simulink model "sschdlexThreePhaseConverterWithGridExample"  (R2023b)
settings: Solver=FixedStepDiscrete  StartTime=0  StopTime=0.09  RelTol=1e-3
InitFcn:
  | % LC filter parameters
  | 
  | Lf = 2e-3;
  | Rf = 20e-3;
  | Cf = 1e-6;
  | 
  | % Sample step size
  | 
  | % if ~exist('Tbase')
  |     Tbase = 5e-9;
  | % end
  | 
  | Ts = 1e-6;
  | Tsc=5e-5;
  | fsw = 10e3;
  | 
  | % PWM oversampling
  | oversampling = Ts/Tbase;
  | 
  | % Frame size for data transfer to CPU
  | frame_size = round(Tsc/Ts);
  | 
  | % Control constants
  | 
  | Kp_id = 1.5;
  | Ki_id = 400;
  | Kp_iq = 1.5;
  | Ki_iq = 400;
libraries: simulink x51, hdlsllib x23, fl_lib x15, nesl_utility x15, slrealtimeloglib x12, ee_lib x11, eeTransforms x3, slpidlib x2, eeSinusoidalMeasurement x1
(part 3 of 3)

== system sschdlexThreePhaseConverterWithGridExample/FPGA/Inverter/Inverter (2-Level HDL w faults)/Calculate Phase Voltage2/Positive Rail Switch Characteristics ==
  Vin : Inport
  I : Inport  Port=2
  Compare To Zero : simulink/Logic and Bit Operations/Compare To Zero  relop=>=  OutDataTypeStr=boolean
  Constant : Constant  Value=vfSwitch  OutDataTypeStr=single  SampleTime=ts_FPGA_mdl
  Constant1 : Constant  Value=vfDiode  OutDataTypeStr=single  SampleTime=ts_FPGA_mdl
  Gain : Gain  Gain=rSwitch
  Gain1 : Gain  Gain=rDiode
  I1 : InportShadow  Port=2
  I2 : InportShadow  Port=2
  Sum1 : Sum  Inputs=-+|
  Sum2 : Sum  Inputs=|++
  Sum3 : Sum  Inputs=+-|
  Switch : Switch  Criteria=u2 > Threshold  SaturateOnIntegerOverflow=off  InputSameDT=off
  Unit Delay : UnitDelay  SampleTime=ts_FPGA_mdl  HasFrameUpgradeWarning=on
  Vout : Outport  VectorParamsAs1DForOutWhenUnconnected=off
  wires:
  Compare To Zero/1 -> Switch/2
  Sum3/1 -> Unit Delay/1
  Sum1/1 -> Switch/3
  I2/1 -> Gain1/1
  Constant1/1 -> Sum1/1
  Gain1/1 -> Sum1/2
  Switch/1 -> Sum3/2
  I1/1 -> Compare To Zero/1
  Vin/1 -> Sum3/1
  Gain/1 -> Sum2/1
  Unit Delay/1 -> Vout/1
  Sum2/1 -> Switch/1
  Constant/1 -> Sum2/2
  I/1 -> Gain/1
